simulink model "absbrake"  (R2020b)
settings: Solver=ode45  StartTime=0.0  StopTime=25  MaxStep=.01  RelTol=1e-3  AbsTol=1e-6
PreLoadFcn:
  | % Load initialization data
  | 
  | sldemo_absdata;
StopFcn:
  | if exist ('sldemo_absbrake_output')
  |   sldemo_absbrakeplots;
  | end
values from neighbouring files (symbols this model uses):
  ctrl = 0    [ModelingAnAntiLockBrakingSystemExample.m]    (also in data.m = 1; sldemo_absdata.m)
  g = 32.18    [data.m]    (also in sldemo_absdata.m)
  m = 50    [data.m]    (also in sldemo_absdata.m)
  mu = [0 .4 .8 .97 1.0 .98 .96 .94 .92 .9 .88 .855 .83 .81 .79 .77 .75 .73 .72 .71 .7]    [data.m]    (also in sldemo_absdata.m)
  Rr = 15/12    (= 1.25)    [data.m]    (also in sldemo_absdata.m)
  slip = (0:.05:1.0)    [data.m]    (also in sldemo_absdata.m)
  v0 = 88    [data.m]    (also in sldemo_absdata.m)
CloseFcn:
  | % Close the plots that are still open
  | h = findobj(0, 'Name', 'ABS Speeds');
  | if ~isempty(h),
  |   close(h);
  | end;
  | 
  | h = findobj(0, 'Name', 'ABS Slip');
  | if ~isempty(h),
  |   close(h);
  | end;
  | 
  | % Clear initial conditions data to avoid cluttering the workspace
  | 
  | clear g v0 Rr Kf m PBmax TB I slip mu ctrl h;
Description:
  | Modeling an Anti-Lock Braking System (ABS)
  | 
  | *Summary*
  | 
  | This example describes a simple model for an Anti-Lock Braking System
  | (ABS). The model simulates the dynamic behavior of a vehicle
  | under hard braking conditions. The model represents a single wheel, which
  | may be replicated a number of times to create a model for a multi-wheel
  | vehicle.
  | 
  | This model uses the signal logging feature in Simulink(R). You log signals to the
  | MATLAB(R) workspace where you can analyze and view them. You can view
  | the code in sldemo_absbrakeplots.m to see how this is done.
  | 
  | In this model, the wheel speed is calculated in a separate component
  | named sldemo_wheelspeed_absbrake.
  | This component is then referenced using a Model block.  Note that both the
  | top model and the referenced model use a variable step solver, so Simulink
  | will track zero-crossings in the referenced model.
settings Model: FPTRunName=Active  ExtModeTrigMode=oneshot  ExtModeArmWhenConnect=off  ExtModeAutoUpdateStatusClock=off  Creator=The MathWorks, Inc.  LastModifiedBy=WELCOME
settings SolverCC: AutoScaleAbsTol=off
settings DataIOCC: SaveFormat=Array  SaveOutput=off  SaveTime=off  ReturnWorkspaceOutputs=off  TimeSaveName=time  SignalLoggingName=sldemo_absbrake_output
settings OptimizationCC: DefaultParameterBehavior=Inlined  InlineInvariantSignals=on  ExpressionDepthLimit=2147483647  InitFltsAndDblsToZero=on  LifeSpan=inf  BufferReusableBoundary=off
settings DebuggingCC: SaveWithParameterizedLinksMsg=none  MultiTaskDSMMsg=warning  SigSpecEnsureSampleTimeMsg=none  IntegerOverflowMsg=none  FcnCallInpInsideContextMsg=warning  BusObjectLabelMismatch=none  AllowSymbolicDim=off  StateNameClashWarn=warning  SFUnexpectedBacktrackingDiag=warning  SFNoUnconditionalDefaultTransitionDiag=warning  SFExecutionAtInitializationDiag=none  IntegerSaturationMsg=none  ArithmeticOperatorsInVariantConditions=warning
settings HardwareCC: ProdBitPerPointer=32  ProdBitPerSizeT=32  ProdBitPerPtrDiffT=32  ProdLargestAtomicFloat=None  ProdIntDivRoundTo=Undefined  ProdEndianess=Unspecified  ProdWordSize=32  ProdHWDeviceType=32-bit Generic  TargetBitPerPointer=64  TargetBitPerSizeT=64  TargetBitPerPtrDiffT=64  TargetLongLongMode=on  TargetIntDivRoundTo=Zero  TargetEndianess=LittleEndian  TargetWordSize=64  TargetHWDeviceType=MATLAB Host
settings ModelReferenceCC: UpdateModelReferenceTargets=IfOutOfDate  PropagateSignalLabelsOutOfModel=off
settings SFSimCC: SimUseLocalCustomCode=off  CustomCodeUndefinedFunction=UseInterfaceOnly
settings RTWCC: RTWUseLocalCustomCode=off
settings CodeAppCC: StateflowObjectComments=on
settings GRTTargetCC: TargetLangStandard=C89/C90 (ANSI)
settings ConfigComp: CovMetricSettings=dw  CovSaveCumulativeToWorkspaceVar=on  CovSaveSingleToWorkspaceVar=on  CovExternalEMLEnable=off  CovSFcnEnable=off

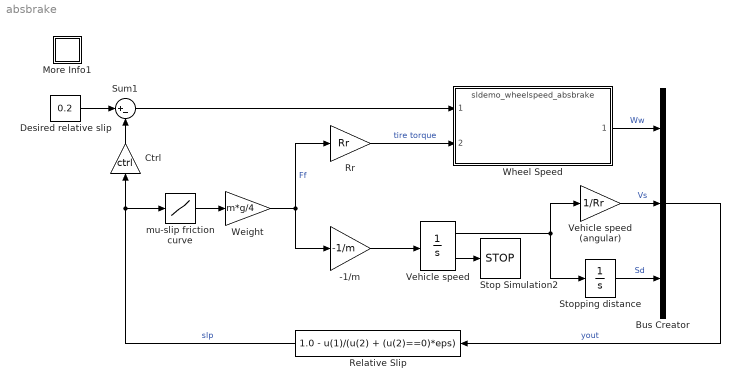
== system absbrake ==
  -1/m : Gain  Gain=-1/m  SaturateOnIntegerOverflow=on  OutDataTypeStr=Inherit: Same as input  ParamDataTypeStr=Inherit: Same as input
  Bus Creator : BusCreator  Inputs=3
  Ctrl : Gain  Gain=ctrl  SaturateOnIntegerOverflow=on  OutDataTypeStr=Inherit: Same as input  ParamDataTypeStr=Inherit: Same as input
  Desired relative slip : Constant  Value=0.2
  More Info1 : Subsystem
      settings: OpenFcn=showExample('simulink_automotive/ModelingAnAntiLockBrakingSystemExample')
      mask Display: disp('?')
  Relative Slip : Fcn  Expr=1.0 - u(1)/(u(2) + (u(2)==0)*eps)
  Rr : Gain  Gain=Rr  SaturateOnIntegerOverflow=on  OutDataTypeStr=Inherit: Same as input  ParamDataTypeStr=Inherit: Same as input
  Stop Simulation2 : Stop
  Stopping distance : Integrator  UpperSaturationLimit=1000  LowerSaturationLimit=0
  Sum1 : Sum  Inputs=|+-  InputSameDT=on  SaturateOnIntegerOverflow=on  OutDataTypeStr=Inherit: Same as first input
  Vehicle speed : Integrator  InitialCondition=v0  LimitOutput=on  UpperSaturationLimit=1000  LowerSaturationLimit=0  ShowSaturationPort=on
  Vehicle speed (angular) : Gain  Gain=1/Rr  SaturateOnIntegerOverflow=on  OutDataTypeStr=Inherit: Same as input  ParamDataTypeStr=Inherit: Same as input
  Weight : Gain  Gain=m*g/4  SaturateOnIntegerOverflow=on  OutDataTypeStr=Inherit: Same as input  ParamDataTypeStr=Inherit: Same as input
  Wheel Speed : ModelReference  ModelNameDialog=sldemo_wheelspeed_absbrake  SimulationMode=Normal  ModelReferenceVersion=1.68
  mu-slip friction curve : Lookup_n-D  NumberOfTableDimensions=1  BreakpointsForDimension1=slip  Table=mu  SaturateOnIntegerOverflow=on  InputSameDT=on
  wires:
  Bus Creator/1 -> Relative Slip/1  "yout"
  Vehicle speed (angular)/1 -> Bus Creator/2  "Vs"
  Relative Slip/1 -> mu-slip friction curve/1, Ctrl/1  "slp"
  Stopping distance/1 -> Bus Creator/3  "Sd"
  -1/m/1 -> Vehicle speed/1
  Vehicle speed/2 -> Stop Simulation2/1
  Vehicle speed/1 -> Stopping distance/1, Vehicle speed (angular)/1
  mu-slip friction curve/1 -> Weight/1
  Weight/1 -> -1/m/1, Rr/1  "Ff"
  Ctrl/1 -> Sum1/2
  Desired relative slip/1 -> Sum1/1
  Sum1/1 -> Wheel Speed/1
  Wheel Speed/1 -> Bus Creator/1  "Ww"
  Rr/1 -> Wheel Speed/2  "tire torque"

== system absbrake/More Info1 ==
